simulink model "MSD_Overall"  (R2022a)
settings: Solver=VariableStepAuto  StartTime=0.0  StopTime=10.0  RelTol=1e-3
model workspace (MAT data in the model file):
  A_CT = [0  1  0  0; -0.3  -2  0.15  0; 0  0  0  1; 0.15  0  -0.15  0]
  B_CT = [0; 0.2; 0; 0]
  C = [0 0 0 1]
  F_in = 1
  Iden = [1  0  0  0; 0  1  0  0; 0  0  1  0; 0  0  0  1]
  K_infty = [2.92191584939e-05; -2.05628372842e-06; 7.30558989491e-09; 0.000936039488485]
  P_k_0 = [0.5  0  0  0; 0  0.5  0  0; 0  0  0.5  0; 0  0  0  0.5]
  Q = 0.01
  R = 0.01
  Ts = 0.1
  b = 10
  k1 = 0.75
  k2 = 0.75
  m1 = 5
  m2 = 5
  x0 = [0; 0; 0; 0]
  x_0_est = [0; 0; 0; 0]
settings Model: Creator=tyevans  LastModifiedBy=tyevans

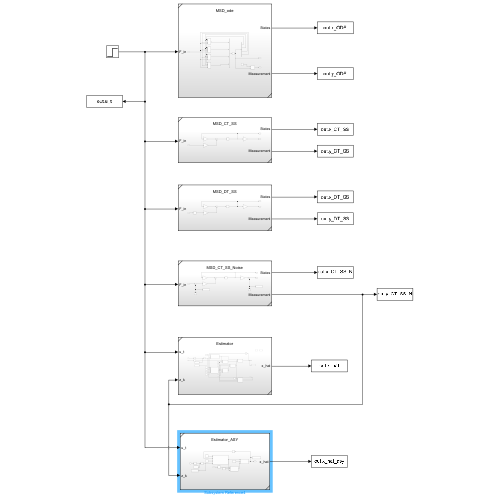
[thumbnail: Simulink's stored preview of the top-level diagram]
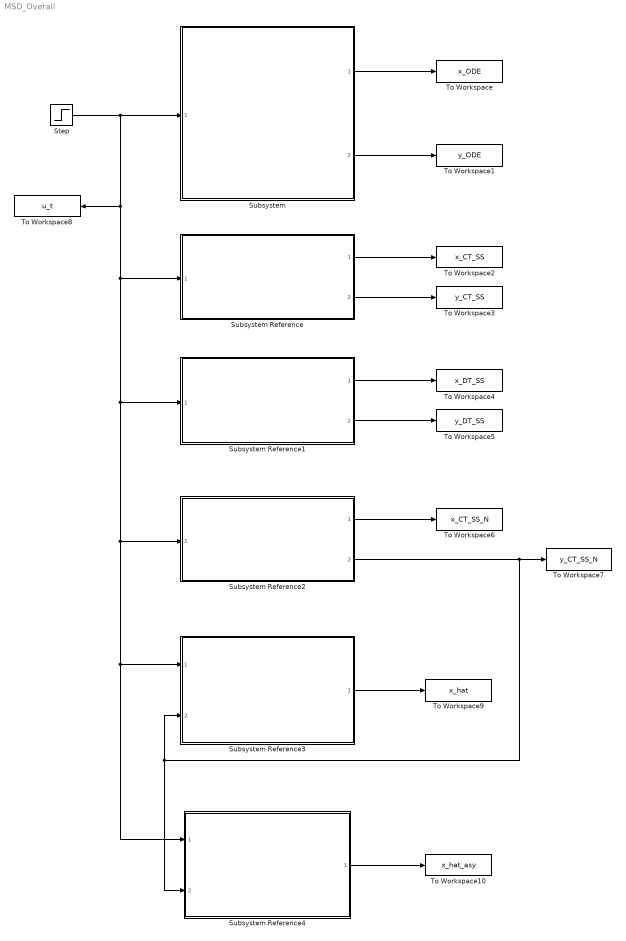
== system MSD_Overall ==
  Step : Step  Time=0  After=F_in  SampleTime=0  VectorParams1D=off
  Subsystem : Subsystem  ReferencedSubsystem=MSD_ode
  Subsystem Reference : Subsystem  ReferencedSubsystem=MSD_CT_SS
  Subsystem Reference1 : Subsystem  ReferencedSubsystem=MSD_DT_SS
  Subsystem Reference2 : Subsystem  ReferencedSubsystem=MSD_CT_SS_Noise
  Subsystem Reference3 : Subsystem  ReferencedSubsystem=Estimator
  Subsystem Reference4 : Subsystem  ReferencedSubsystem=Estimator_ASY
  To Workspace : ToWorkspace  VariableName=x_ODE  SaveFormat=Structure With Time  SampleTime=-1
  To Workspace1 : ToWorkspace  VariableName=y_ODE  SaveFormat=Structure With Time  SampleTime=-1
  To Workspace10 : ToWorkspace  VariableName=x_hat_asy  SaveFormat=Structure With Time  SampleTime=-1
  To Workspace2 : ToWorkspace  VariableName=x_CT_SS  SaveFormat=Structure With Time  SampleTime=-1
  To Workspace3 : ToWorkspace  VariableName=y_CT_SS  SaveFormat=Structure With Time  SampleTime=-1
  To Workspace4 : ToWorkspace  VariableName=x_DT_SS  SaveFormat=Structure With Time  SampleTime=-1
  To Workspace5 : ToWorkspace  VariableName=y_DT_SS  SaveFormat=Structure With Time  SampleTime=-1
  To Workspace6 : ToWorkspace  VariableName=x_CT_SS_N  SaveFormat=Structure With Time  SampleTime=-1
  To Workspace7 : ToWorkspace  VariableName=y_CT_SS_N  SaveFormat=Structure With Time  SampleTime=-1
  To Workspace8 : ToWorkspace  VariableName=u_t  SaveFormat=Structure With Time  SampleTime=-1
  To Workspace9 : ToWorkspace  VariableName=x_hat  SaveFormat=Structure With Time  SampleTime=-1
  wires:
  Subsystem/1 -> To Workspace/1
  Subsystem/2 -> To Workspace1/1
  Subsystem Reference/1 -> To Workspace2/1
  Subsystem Reference/2 -> To Workspace3/1
  Subsystem Reference1/1 -> To Workspace4/1
  Subsystem Reference1/2 -> To Workspace5/1
  Subsystem Reference2/1 -> To Workspace6/1
  Subsystem Reference3/1 -> To Workspace9/1
  Step/1 -> To Workspace8/1, Subsystem Reference4/1, Subsystem Reference3/1, Subsystem Reference2/1, Subsystem Reference1/1, Subsystem Reference/1, Subsystem/1
  Subsystem Reference2/2 -> Subsystem Reference4/2, Subsystem Reference3/2, To Workspace7/1
  Subsystem Reference4/1 -> To Workspace10/1
